simulink model "pmsm_model_project"  (R2023a)
settings: Solver=ode23tb  StartTime=0.0  StopTime=Tf  FixedStep=Tsim  MaxStep=Tsim  MinStep=Tsim/100  RelTol=1e-3
values from neighbouring files (symbols this model uses):
  A = 0.1    [pmsm_param_project.m]
  C32 = [ 1       0 ... (first row only)    [pmsm_param_project.m]
  C32inv = 2/3*[1    -1/2        -1/2 ... (first row only)    [pmsm_param_project.m]
  C33 = C32*C32inv    [pmsm_param_project.m]
  Cb = 500e-6    (= 0.0005)    [pmsm_param_project.m]
  dTm0 = 0.20*Tmrated    (= 48)    [pmsm_param_project.m]
  Dyno = 1    [pmsm_param_project.m]
  f = 15e-3    (= 0.015)    [pmsm_param_project.m]
  GVSI = 1    [pmsm_param_project.m]
  Id0 = interp1(Tref,Idopt,Tm0)    [pmsm_param_project.m]
  Idc0 = Pe0/VDC    [pmsm_param_project.m]
  Idopt = zeros(1,NT)    [pmsm_param_project.m]
  Iq0 = interp1(Tref,Iqopt,Tm0)    [pmsm_param_project.m]
  Iqopt = zeros(1,NT)    [pmsm_param_project.m]
  J = 100e-3    (= 0.1)    [pmsm_param_project.m]
  Kid = Kpd/tid    (= -180)    [pmsm_param_project.m]
  Kiq = Kpq/tiq    (= -180)    [pmsm_param_project.m]
  kL = 0.750    (= 0.75)    [pmsm_param_project.m]
  Kpd = -3*Ld0/tr    (= -3)    [pmsm_param_project.m]
  Kpq = -3*Lq0/tr    (= -6)    [pmsm_param_project.m]
  Lb = 20e-6    (= 2e-05)    [pmsm_param_project.m]
  Ld0 = 1.0*Ld    (= 0.001)    [pmsm_param_project.m]
  Lq0 = 1.0*Lq    (= 0.002)    [pmsm_param_project.m]
  Pe0 = 3/2*(Vd0*Id0+Vq0*Iq0)    [pmsm_param_project.m]
  Pp = 4    [pmsm_param_project.m]
  Psid0 = interpn(Idv,Iqv,Psidd,Id0,Iq0)    [pmsm_param_project.m]
  Psif0 = 1.0*Psif    (= 0.167)    [pmsm_param_project.m]
  Psiq0 = interpn(Idv,Iqv,Psiqq,Id0,Iq0)    [pmsm_param_project.m]
  Qbat = 72*3600    (= 259200)    [pmsm_param_project.m]
  RateTm = 10000    [pmsm_param_project.m]
  rb = 80e-3    (= 0.08)    [pmsm_param_project.m]
  Rs = 60e-3    (= 0.06)    [pmsm_param_project.m]
  Rs0 = 1.0*Rs    (= 0.06)    [pmsm_param_project.m]
  SOC0 = 0.50    (= 0.5)    [pmsm_param_project.m]
  Thetae0 = 0    [pmsm_param_project.m]
  Tm0 = (kL+f)*Wm0    (= 192.2654704)    [pmsm_param_project.m]
  Tp = 200e-6    (= 0.0002)    [pmsm_param_project.m]
  Tref = -Tmax:Tmax/100:Tmax    [pmsm_param_project.m]
  Ts = Tp    (= 0.0002)    [pmsm_param_project.m]
  Tsim = min([Tp Ts])/100    [pmsm_param_project.m]
  TSS = Tstep+0.050    (= 0.1)    [pmsm_param_project.m]
  Tstep = 0.050    (= 0.05)    [pmsm_param_project.m]
  Ud0 = Rs*Id0    (= 0)    [pmsm_param_project.m]
  Uq0 = Rs*Iq0    (= 11.5129024191)    [pmsm_param_project.m]
  Vd0 = Ud0-Pp*Psiq0*Wm0    [pmsm_param_project.m]
  VDC = 800    [pmsm_param_project.m]
  VDC0 = 0.8*VDC    (= 640)    [pmsm_param_project.m]
  Vp = VDC/2    (= 400)    [pmsm_param_project.m]
  Vq0 = Uq0+Pp*Psid0*Wm0    [pmsm_param_project.m]
  wh = 10000    [pmsm_param_project.m]
  Wm0 = 2400*pi/30    (= 251.327412287)    [pmsm_param_project.m]
undefined symbols (not defined in the file or in its folder): fdesignblkfcn, gcbh, Idd, Idrop, Iqq, Isw, Psidv, Psiqv, SwLoss, Vdrop
libraries: simulink x11, slpidlib x1, dspfdesign x1, spsTHDLib x1
(part 2 of 2)

== system pmsm_model_project/VSI/VSI_Power/Subsystem1/Derivative ==
  E : Inport
  Divide1 : Product  Inputs=/*
  Saturation : Saturate  UpperLimit=inf  LowerLimit=1e-9
  Sum2 : Sum  Inputs=|+-
  Sum5 : Sum  Inputs=+-|
  Unit Delay1 : UnitDelay  SampleTime=-1  HasFrameUpgradeWarning=on
  Unit Delay2 : UnitDelay  SampleTime=-1  HasFrameUpgradeWarning=on
  P : Outport
  wires:
  Unit Delay2/1 -> Sum5/2
  Saturation/1 -> Divide1/1
  [Clk] -> Sum5/1, Unit Delay2/1
  E/1 -> Unit Delay1/1, Sum2/1
  Unit Delay1/1 -> Sum2/2
  Sum5/1 -> Saturation/1
  Sum2/1 -> Divide1/2
  Divide1/1 -> P/1

== system pmsm_model_project/VSI/VSI_Power/Subsystem1/Subsystem1 ==
  U : Inport
  Gain : Gain
  Gain1 : Gain
  Subsystem : Subsystem
  Subsystem1 : Subsystem
  Sum3 : Sum  Inputs=|++  SaturateOnIntegerOverflow=on
  Out1 : Outport
  wires:
  U/1 -> Subsystem/1(U), Subsystem1/1(U)
  Subsystem1/1(Out1) -> Gain1/1
  Subsystem/1(Out1) -> Gain/1
  Gain/1 -> Sum3/2
  Sum3/1 -> Out1/1
  Gain1/1 -> Sum3/1

== system pmsm_model_project/VSI/VSI_Power/Subsystem1/Subsystem2 ==
  U : Inport
  Gain : Gain
  Gain1 : Gain
  Subsystem : Subsystem
  Subsystem1 : Subsystem
  Sum3 : Sum  Inputs=|++  SaturateOnIntegerOverflow=on
  Out1 : Outport
  wires:
  Gain1/1 -> Sum3/1
  Sum3/1 -> Out1/1
  Gain/1 -> Sum3/2
  Subsystem/1(Out1) -> Gain/1
  Subsystem1/1(Out1) -> Gain1/1
  U/1 -> Subsystem1/1(U), Subsystem/1(U)

== system pmsm_model_project/VSI/VSI_Power/Subsystem1/Subsystem3 ==
  U : Inport
  Gain : Gain
  Gain1 : Gain
  Subsystem : Subsystem
  Subsystem1 : Subsystem
  Sum3 : Sum  Inputs=|++  SaturateOnIntegerOverflow=on
  Out1 : Outport
  wires:
  Gain1/1 -> Sum3/1
  Sum3/1 -> Out1/1
  Gain/1 -> Sum3/2
  Subsystem/1(Out1) -> Gain/1
  Subsystem1/1(Out1) -> Gain1/1
  U/1 -> Subsystem1/1(U), Subsystem/1(U)

== system pmsm_model_project/VSI/VSI_Power/Subsystem1/Sum  ==
  x : Inport
  Memory : Memory
  Sum1 : Sum  Inputs=|++
  Sx : Outport
  wires:
  Memory/1 -> Sum1/2
  x/1 -> Sum1/1
  Sum1/1 -> Memory/1, Sx/1

== system pmsm_model_project/VSI/VSI_Power/Subsystem1/Subsystem1/Subsystem ==
  U : Inport
  Compare To Constant : simulink/Logic and Bit Operations/Compare To Constant  relop=<  const=-VDC0  OutDataTypeStr=uint8
  Memory : Memory
  Sum : Sum  Inputs=+-|
  Out1 : Outport
  wires:
  Compare To Constant/1 -> Out1/1
  U/1 -> Sum/1, Memory/1
  Sum/1 -> Compare To Constant/1
  Memory/1 -> Sum/2

== system pmsm_model_project/VSI/VSI_Power/Subsystem1/Subsystem1/Subsystem1 ==
  U : Inport
  Compare To Constant : simulink/Logic and Bit Operations/Compare To Constant  relop=>  const=VDC0  OutDataTypeStr=uint8
  Memory : Memory
  Sum : Sum  Inputs=+-|
  Out1 : Outport
  wires:
  Compare To Constant/1 -> Out1/1
  Memory/1 -> Sum/2
  Sum/1 -> Compare To Constant/1
  U/1 -> Sum/1, Memory/1

== system pmsm_model_project/VSI/VSI_Power/Subsystem1/Subsystem2/Subsystem ==
  U : Inport
  Compare To Constant : simulink/Logic and Bit Operations/Compare To Constant  relop=<  const=-VDC0  OutDataTypeStr=uint8
  Memory : Memory
  Sum : Sum  Inputs=+-|
  Out1 : Outport
  wires:
  Memory/1 -> Sum/2
  Sum/1 -> Compare To Constant/1
  U/1 -> Memory/1, Sum/1
  Compare To Constant/1 -> Out1/1

== system pmsm_model_project/VSI/VSI_Power/Subsystem1/Subsystem2/Subsystem1 ==
  U : Inport
  Compare To Constant : simulink/Logic and Bit Operations/Compare To Constant  relop=>  const=VDC0  OutDataTypeStr=uint8
  Memory : Memory
  Sum : Sum  Inputs=+-|
  Out1 : Outport
  wires:
  U/1 -> Memory/1, Sum/1
  Sum/1 -> Compare To Constant/1
  Memory/1 -> Sum/2
  Compare To Constant/1 -> Out1/1

== system pmsm_model_project/VSI/VSI_Power/Subsystem1/Subsystem3/Subsystem ==
  U : Inport
  Compare To Constant : simulink/Logic and Bit Operations/Compare To Constant  relop=<  const=-VDC0  OutDataTypeStr=uint8
  Memory : Memory
  Sum : Sum  Inputs=+-|
  Out1 : Outport
  wires:
  Memory/1 -> Sum/2
  Sum/1 -> Compare To Constant/1
  U/1 -> Memory/1, Sum/1
  Compare To Constant/1 -> Out1/1

== system pmsm_model_project/VSI/VSI_Power/Subsystem1/Subsystem3/Subsystem1 ==
  U : Inport
  Compare To Constant : simulink/Logic and Bit Operations/Compare To Constant  relop=>  const=VDC0  OutDataTypeStr=uint8
  Memory : Memory
  Sum : Sum  Inputs=+-|
  Out1 : Outport
  wires:
  U/1 -> Memory/1, Sum/1
  Sum/1 -> Compare To Constant/1
  Memory/1 -> Sum/2
  Compare To Constant/1 -> Out1/1

== matlab function pmsm_model_project/PMSM/dq-PMSM ==
  data: vd input; dPsid output; vq input; id input; iq input; Psid input; Psiq input; Omega input; TL input; dPsiq output; dOmega output; dTheta output; Rs input; Pp parameter; f parameter; J parameter; Tm output
function [dPsid, dPsiq, dOmega, dTheta, Tm] = PMSM(vd, vq, id, iq, Psid, Psiq, Omega, TL, Rs, Pp, f, J)

w=Pp*Omega;
Tm=(3/2)*Pp*(Psid*iq-Psiq*id);   % Clarke
% Tm=p*(Psid*iq-Psiq*id);       % Concordia

dPsid=vd-Rs*id+w*Psiq;
dPsiq=vq-Rs*iq-w*Psid;
dOmega=(Tm-f*Omega-TL)/J;
dTheta=w;

== matlab function pmsm_model_project/Control/Ctrl ==
  data: method input; idref input; idm input; iqref input; iqm input; we input; VDC input; Pp parameter; Psif0 parameter; Ld0 parameter; Lq0 parameter; Rs0 parameter; Ts parameter; vd output; vq output; Kpd parameter; Kpq parameter; Kid parameter; Kiq parameter; Id0 parameter; Iq0 parameter; Ud0 parameter; Uq0 parameter; Tm0 parameter; Vd0 parameter; Vq0 parameter; load output; Rs input
function [vd, vq, load]  = Ctrl(method, idref, idm, iqref, iqm, we, VDC, Pp, Psif0, Ld0, Lq0, Rs0, Ts, Kpd, Kpq, Kid, Kiq, Id0, Iq0, Ud0, Uq0, Tm0, Vd0, Vq0, Rs)

persistent interrd interrq exetime

method=fix(method);
if method<0, method=0; end
if method>9, method=9; end

if isempty(interrd), if method==0, interrd = Vd0; else interrd = Ud0; end, end
if isempty(interrq), if method==0, interrq = Vq0; else interrq = Uq0; end, end
if isempty(exetime), exetime = 0; end

tic

switch method
    case 0   % PI
        errd=idref-idm;
        errq=iqref-iqm;
        interrd=interrd+Kid*errd*Ts;
        interrq=interrq+Kiq*errq*Ts;
        vd=Kpd*errd+interrd;
        vq=Kpq*errq+interrq;
    case 1   % PI+feedback decoupling
        errd=idref-idm;
        errq=iqref-iqm;
        interrd=interrd+Kid*errd*Ts;
        interrq=interrq+Kiq*errq*Ts;
        vd=Kpd*errd+interrd-Lq0*iqm*we;
        vq=Kpq*errq+interrq+(Psif0+Ld0*idm)*we;

        Vs = sqrt(vd^2 + vq^2);
        Vmax = VDC / sqrt(3);
        if (Vs > Vmax)

            vd = vd*(Vmax)/Vs;
            vq = vq*(Vmax)/Vs;
        end
    case 2   % Deadbeat MPC
        vd=Rs0*idm - we*Lq0*iqm + Ld0/Ts*(idref - idm) + Kpd*(idref - idm);
        vq=Rs0*iqm + we*(Ld0*idm + Psif0) + Lq0/Ts*(iqref - iqm) + Kpq*(iqref - iqm);     
        Vs = sqrt(vd^2 + vq^2);
        Vmax = VDC / sqrt(3);
        if (Vs > Vmax)

            vd = vd*Vmax/Vs;
            vq = vq*Vmax/Vs;
        end
    case 3   % CCS-MPC + decoupling + gradient?
        vd=0;
        vq=0;       
    otherwise
        vd=0;
        vq=0;
end

exetime=exetime+toc;
load=exetime;
